simulink model "matrix_multiply_test"  (R2018a)
settings: Solver=VariableStepAuto  StartTime=0.0  StopTime=10.0  RelTol=1e-3
libraries: modelsimlib x1
settings Model: Creator=paull  LastModifiedBy=paull

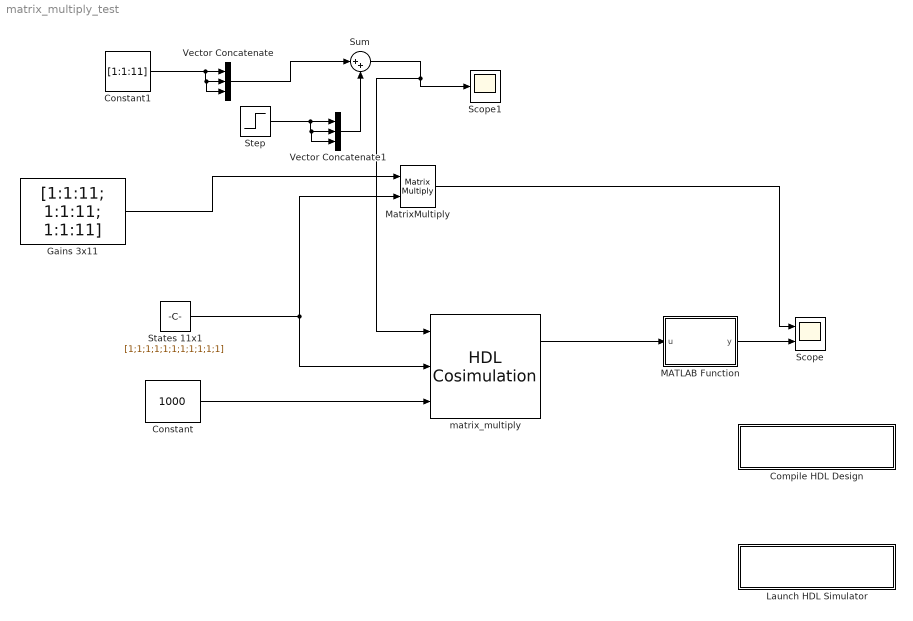
== system matrix_multiply_test ==
  Compile HDL Design : Subsystem
      settings: OpenFcn=eval('compile_hdl_design_matrix_multiply');
      mask Display: disp(['Double-Click to' char(10) 'compile HDL files'])
  Constant : Constant  Value=1000  OutDataTypeStr=uint32
  Constant1 : Constant  Value=[1:1:11]
  Gains 3x11 : Constant  Value=[1:1:11; 1:1:11; 1:1:11]  VectorParams1D=off  OutDataTypeStr=double
  Launch HDL Simulator : Subsystem
      settings: OpenFcn=eval('launch_hdl_simulator_matrix_multiply');
      mask Display: disp(['Double-Click to' char(10) 'launch HDL simulator'])
  MATLAB Function : MATLAB Function  TreatAsAtomicUnit=on
  MatrixMultiply : Product  Multiplication=Matrix(*)
  Scope : Scope  NumInputPorts=2
  Scope1 : Scope
  States 11x1 : Constant  Value=[1;1;1;1;1;1;1;1;1;1;1]  OutDataTypeStr=double
  Step : Step  Time=5  Before=[0 0 0 0 0 0 0 0 0 0 0]  After=[1:1:11]
  Sum : Sum  Inputs=|++
  Vector Concatenate : Concatenate  NumInputs=3
  Vector Concatenate1 : Concatenate  NumInputs=3
  matrix_multiply : modelsimlib/HDL Cosimulation  PortPaths=/matrix_multiply/input_gains_matrix;/matrix_multiply/input_states_matrix;/matrix_multiply/sample_time;/matrix_multiply/output_matrix;/matrix_multiply/output_valid;  PortModes=[1 1 1 2 2 ]  PortTimes=[-1,-1,-1,1,1]  PortSigns=[-1,-1,-1,-1,-1,]  PortFracLengths=[0,0,0,0,0]  CommLocal=on  CommSharedMemory=on  CommPortNumber=4449  CommShowInfo=on  ClockModes=[]  ClockTimes=[]  TclPreSimCommand=|  TclPostSimCommand=|  TimingMode=ns  TimingScaleFactor=1e4  idxCellArray={'UNUSED_VAR'}  CosimBypass=Full Simulation  AllowDirectFeedthrough=on  ProductName=EDA Simulator Link MQ  RunAutoTimescale=off  HdlClocks=/matrix_multiply/clock 10 ns;  PreRunTime=10  PreRunTimeUnit=ns
      TclPreSimCommand=|
      | force /matrix_multiply/clock 0 0 ns, 1 5 ns -repeat 10 ns;
      | force /matrix_multiply/reset 1 0 ns, 0 8 ns;
      TclPostSimCommand=|
      | noforce /matrix_multiply/clock;
      | noforce /matrix_multiply/reset;
      | puts "done";
      settings: SourceProductName=HDL Verifier  SourceProductBaseCode=ES
  wires:
  Constant/1 -> matrix_multiply/3
  matrix_multiply/1 -> MATLAB Function/1(u)
  MATLAB Function/1(y) -> Scope/2
  MatrixMultiply/1 -> Scope/1
  States 11x1/1 -> matrix_multiply/2, MatrixMultiply/2
  Constant1/1 -> Vector Concatenate/3, Vector Concatenate/2, Vector Concatenate/1
  Gains 3x11/1 -> MatrixMultiply/1
  Step/1 -> Vector Concatenate1/3, Vector Concatenate1/2, Vector Concatenate1/1
  Vector Concatenate/1 -> Sum/1
  Vector Concatenate1/1 -> Sum/2
  Sum/1 -> matrix_multiply/1, Scope1/1

== system matrix_multiply_test/Compile HDL Design ==

== system matrix_multiply_test/Launch HDL Simulator ==

== matlab function matrix_multiply_test/MATLAB Function ==
  data: u input double size=3; y output double size=3
function y = fcn(u)

y = u;
